simulink model "temp_m"  (R2018b)
settings: Solver=FixedStepAuto  StartTime=0.0  StopTime=14.5  FixedStep=0.1  RelTol=1e-3
settings Model: Creator=beniamin.costandin  LastModifiedBy=beniamin.costandin

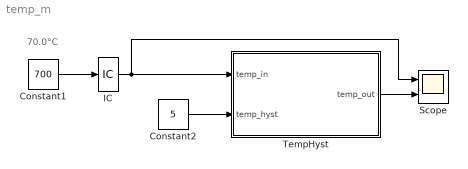
== system temp_m ==
  note: 70.0°C
  Constant1 : Constant  Value=700
  Constant2 : Constant  Value=5  OutDataTypeStr=uint16
  IC : InitialCondition  Value=0
  Scope : Scope  NumInputPorts=2
  TempHyst : MATLAB Function  TreatAsAtomicUnit=on
  wires:
  Constant1/1 -> IC/1
  IC/1 -> Scope/1, TempHyst/1(temp_in)
  TempHyst/1(temp_out) -> Scope/2
  Constant2/1 -> TempHyst/2(temp_hyst)

== matlab function temp_m/TempHyst ==
  data: temp_out output; temp_in input; temp_hyst input
function temp_out = fcn(temp_in,temp_hyst)

persistent temp_out_prev;
temp_diff = uint16(0);

if isempty(temp_out_prev)
    temp_out_prev = uint16(temp_in); 
end

%check if temperature is rising
if (temp_in > temp_out_prev)
    %calculate the difference between t_in and t_out
    temp_diff = temp_in - temp_out_prev;
    
    if (temp_diff >= temp_hyst)
        %increase output with one hyst value
        temp_out_prev = temp_out_prev + uint16(temp_hyst);
    end


%check if the temperature is decreasing
elseif (temp_in < temp_out_prev)
    %calculate the difference between t_out and t_in
    temp_diff = temp_out_prev - temp_in;
    
    if (temp_diff >= temp_hyst)
        %decrease output one hyst value
        temp_out_prev = temp_out_prev - uint16(temp_hyst);
    end
    
end

temp_out = temp_out_prev;
